simulink model "controller2"  (R2019a)
settings: Solver=VariableStepAuto  StartTime=0.0  StopTime=2  RelTol=1e-3
values from neighbouring files (symbols this model uses):
  Kd1 = 45    [ILC2dof.m]    (also in PD2dof.m = 42)
  Kd2 = 20    [ILC2dof.m]    (also in PD2dof.m = 8)
  Kp1 = 100    [ILC2dof.m]    (also in PD2dof.m = 1000)
  Kp2 = 40    [ILC2dof.m]    (also in PD2dof.m = 1000)
settings Model: Creator=Simone  LastModifiedBy=simone
settings DataIOCC: ReturnWorkspaceOutputs=off
settings DebuggingCC: ArithmeticOperatorsInVariantConditions=warning

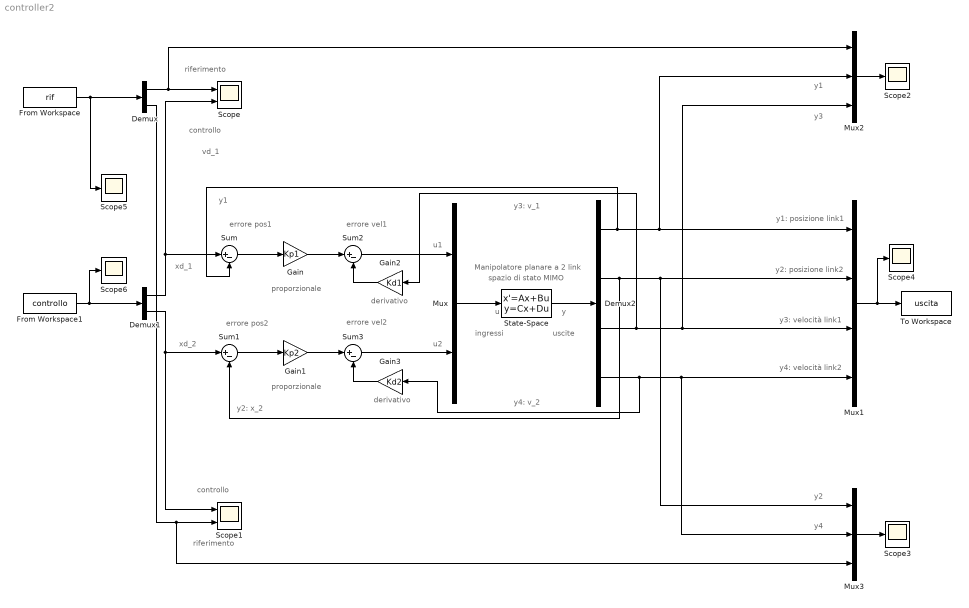
== system controller2 ==
  note: xd_1
  note: derivativo
  note: ingressi
  note: Manipolatore planare a 2 link
  note: spazio di stato MIMO
  note: y3: v_1
  note: y2
  note: xd_2
  note: y4
  note: y1: posizione link1
  note: controllo
  note: y
  note: u
  note: vd_1
  note: u2
  note: y2: posizione link2
  note: u1
  note: uscite
  note: controllo
  note: errore pos1
  note: riferimento
  note: errore vel2
  note: derivativo
  note: y1
  note: proporzionale
  note: y3: velocità link1
  note: y3
  note: riferimento
  note: errore pos2
  note: y4: velocità link2
  note: y1
  note: y4: v_2
  note: errore vel1
  note: y2: x_2
  note: proporzionale
  Demux : Demux  Outputs=2
  Demux1 : Demux  Outputs=2
  Demux2 : Demux
  From Workspace : FromWorkspace  VariableName=rif  SampleTime=0
  From Workspace1 : FromWorkspace  VariableName=controllo  SampleTime=0
  Gain : Gain  Gain=Kp1
  Gain1 : Gain  Gain=Kp2
  Gain2 : Gain  Gain=Kd1
  Gain3 : Gain  Gain=Kd2
  Mux : Mux  Inputs=2
  Mux1 : Mux
  Mux2 : Mux  Inputs=3
  Mux3 : Mux  Inputs=3
  Scope : Scope  NumInputPorts=2
  Scope1 : Scope  NumInputPorts=2
  Scope{2..6} (5 alike) : Scope
  State-Space : StateSpace  A=[0 0 1 0; 0 0 0 1; 0 0 0 0; 0 0 0 0]  B=|  C=[1 0 0 0; 0 1 0 0; 0 0 1 0; 0 0 0 1]  D=[0 0 ; 0 0 ; 0 0; 0 0]  InitialCondition=[1.908103808224664; -1.318116071652818; 0; 0]
      | [0 0 ; 0 0 ; 1.7143  -4.2857; -4.2857  13.7143
      | ]
  Sum{,1..3} (4 alike) : Sum  Inputs=|+-
  To Workspace : ToWorkspace  VariableName=uscita  SaveFormat=Structure With Time  SampleTime=0.01
  wires:
  Demux/2 -> Scope1/2, Mux3/3
  Sum3/1 -> Mux/2
  Sum/1 -> Gain/1
  Demux1/2 -> Scope1/1, Sum1/1
  Mux/1 -> State-Space/1
  Demux2/2 -> Mux3/1, Mux1/2, Sum1/2
  Demux2/1 -> Mux2/2, Mux1/1, Sum/2
  Demux2/4 -> Gain3/1, Mux3/2, Mux1/4
  Sum1/1 -> Gain1/1
  Mux3/1 -> Scope3/1
  Gain3/1 -> Sum3/2
  Gain/1 -> Sum2/1
  Demux2/3 -> Gain2/1, Mux2/3, Mux1/3
  Mux2/1 -> Scope2/1
  Gain1/1 -> Sum3/1
  From Workspace/1 -> Scope5/1, Demux/1
  From Workspace1/1 -> Scope6/1, Demux1/1
  Gain2/1 -> Sum2/2
  State-Space/1 -> Demux2/1
  Mux1/1 -> To Workspace/1, Scope4/1
  Sum2/1 -> Mux/1
  Demux/1 -> Mux2/1, Scope/1
  Demux1/1 -> Scope/2, Sum/1
